simulink model "problem2"  (R2020b)
settings: Solver=VariableStepAuto  StartTime=0.0  StopTime=10.0  RelTol=1e-3
libraries: SignalEditorBlockLib x1
settings Model: Creator=admin  LastModifiedBy=admin

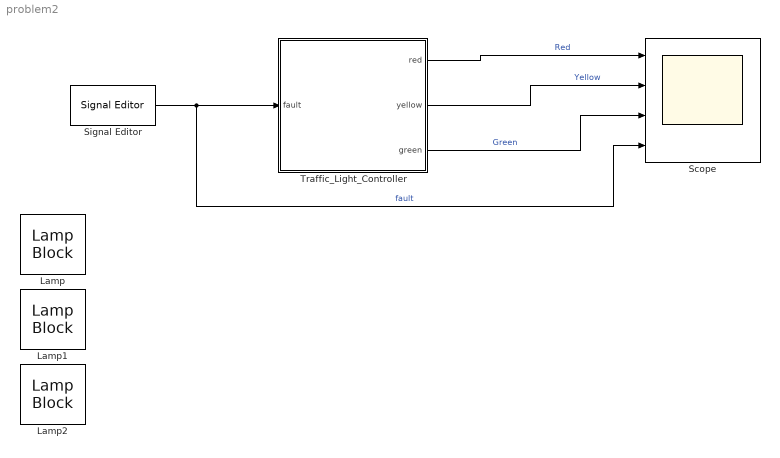
== system problem2 ==
  Lamp : LampBlock
  Lamp1 : LampBlock
  Lamp2 : LampBlock
  Scope : Scope  NumInputPorts=4
  Signal Editor : SignalEditorBlockLib/Signal Editor  FileName=trafficLightFault.mat  ActiveScenario=Faults  ActiveSignal=fault  IsBus=off  OutputBusObjectStr=Bus: BusObject  SampleTime=1  Interpolate=off  ZeroCross=off  OutputAfterFinalValue=Setting to zero  Unit=inherit  PreserveSignalName=on
  Traffic_Light_Controller : Stateflow chart  TreatAsAtomicUnit=on
  wires:
  Traffic_Light_Controller/3(green) -> Scope/3  "Green"
  Signal Editor/1 -> Scope/4, Traffic_Light_Controller/1(fault)  "fault"
  Traffic_Light_Controller/2(yellow) -> Scope/2  "Yellow"
  Traffic_Light_Controller/1(red) -> Scope/1  "Red"

== stateflow chart problem2/Traffic_Light_Controller ==
  state Normal
    state Stop
      % Red light
      entry:
      red = 1;
      yellow = 0;
      green = 0;
    state PrepareToStop
      % Yellow light
      entry:
      red = 0;
      yellow = 1;
      green = 0;
    state Go
      % Green light
      entry:
      red = 0;
      yellow = 0;
      green = 1;
    (default) -> Stop
    Stop -> (junction 11)
    (junction 11) -> (junction 1) : after(3,sec)
    PrepareToStop -> Stop : after(3,sec)
    Go -> PrepareToStop : after(10,sec)
    (junction 1) -> Go
  state Fault
    entry:
    yellow = 0;
    green = 0;
    state BlinkOn
      % Red light
      entry:
      red = 1;
    state BlinkOff
      % No light
      entry:
      red = 0;
    (default) -> BlinkOn
    BlinkOff -> BlinkOn : after(1,sec)
    BlinkOn -> BlinkOff : after(1,sec)
  (default) -> Normal
  Normal -> Fault : [fault == 1]
  Fault -> Normal : [fault == 0]
  data: fault input; red output; yellow output; green output
